simulink library "phasedenvlib"  (R2018b)
settings: Solver=ode45  StartTime=0.0  StopTime=10.0  RelTol=1e-3  EnableMultiTasking=on
undefined symbols (not defined in the file or in its folder): azelaxes, phased, physconst
settings Model: Creator=The MathWorks, Inc.  LastModifiedBy=The MathWorks, Inc.
settings DataIOCC: LimitDataPoints=on  SaveFormat=Array
settings OptimizationCC: LifeSpan=inf
settings DebuggingCC: UnderspecifiedInitializationDetection=Classic  MergeDetectMultiDrivingBlocksExec=none  SolverPrmCheckMsg=warning  AllowSymbolicDim=off  SFUnexpectedBacktrackingDiag=warning  SFNoUnconditionalDefaultTransitionDiag=warning  SFExecutionAtInitializationDiag=none
settings HardwareCC: ProdBitPerPointer=32  ProdBitPerSizeT=32  ProdBitPerPtrDiffT=32  ProdLargestAtomicFloat=None  ProdIntDivRoundTo=Undefined  ProdEndianess=Unspecified  ProdWordSize=32  ProdHWDeviceType=32-bit Generic
settings ModelReferenceCC: PropagateSignalLabelsOutOfModel=off
settings SFSimCC: SimUseLocalCustomCode=off
settings RTWCC: RTWUseLocalCustomCode=off
settings CodeAppCC: StateflowObjectComments=on
settings GRTTargetCC: TargetLangStandard=C89/C90 (ANSI)  GeneratePreprocessorConditionals=Disable all
settings ConfigComp: CovMetricSettings=dw  CovHtmlReporting=on  CovSaveCumulativeToWorkspaceVar=on  CovSaveSingleToWorkspaceVar=on  CovShowResultsExplorer=off  CovExternalEMLEnable=off  CovSFcnEnable=off

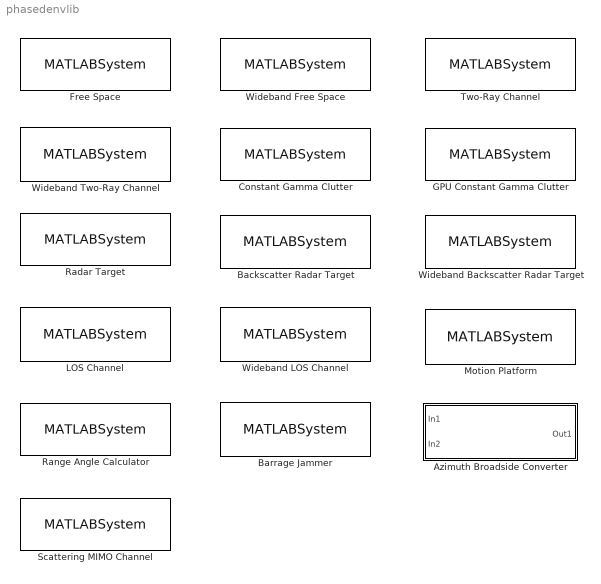
== system phasedenvlib ==
  Azimuth Broadside Converter : Subsystem  VariantControlMode=Label  Variant=on  LabelModeActiveChoice=AzimuthToBroadside  mask(Azimuth/broadside converter){Mode=azimuth -> broadside}
      mask prompts: Mode "Conversion mode:"
      mask help: Conversion between azimuth and broadside angles.
      mask init:
      | modestr = get_param(gcb,'Mode');
      | if modestr(1) == 'a'
      |     mvarctrl = 'AzimuthToBroadside';
      |     inportlabel = 'az';
      |     outportlabel = 'bsd';
      |     titlestr = 'az->bsd';
      | else
      |     mvarctrl = 'BroadsideToAzimuth';
      |     inportlabel = 'bsd';
      |     outportlabel = 'az';
      |     titlestr = 'bsd->az';
      | end
      | set_param(gcb, 'OverrideUsingVariant', mvarctrl);
      mask TypeOptions Mode: azimuth -> broadside | broadside -> azimuth
      mask Display:
      | port_label('input',1,inportlabel);
      | port_label('input',2,'el');
      | port_label('output',1,outportlabel);
      | fprintf('%s',titlestr)
  Backscatter Radar Target : MATLABSystem  System=phased.BackscatterRadarTarget  EnablePolarization=off  AzimuthAngles=-180:180  ElevationAngles=-90:90  RCSPattern=ones(181,361)  ShhPattern=ones(181,361)  ShvPattern=ones(181,361)  SvvPattern=ones(181,361)  Model=Nonfluctuating  PropagationSpeed=physconst( 'LightSpeed' )  OperatingFrequency=3e8  SeedSource=Property  Seed=randi(65535,1)  SimulateUsing=Interpreted execution
      mask Type: phased.BackscatterRadarTarget
      mask Display:
      | disp(['Backscatter' char(10) ' Target']);
      | port_label('input',1,'X');
      | port_label('input',2,'Ang');
  Barrage Jammer : MATLABSystem  System=phased.internal.SimulinkBarrageJammer  ERP=5000  SamplesPerFrameSource=Property  SamplesPerFrame=100  SeedSource=Property  Seed=randi(65535,1)  SimulateUsing=Interpreted execution
      mask Type: phased.internal.SimulinkBarrageJammer
      mask Display: disp('Barrage');
  Constant Gamma Clutter : MATLABSystem  System=phased.internal.SimulinkConstantGammaClutter  Gamma=0  EarthModel=Flat  MaximumRange=5000  AzimuthCoverage=60  PatchAzimuthWidth=1  CoherenceTime=inf  PropagationSpeed=physconst( 'LightSpeed' )  SampleRate=1e6  PRF=1e4  PRFSelectionInputPort=off  SimulationTimeSource=Derive from waveform parameters  OutputFormat=Pulses  NumPulses=1  NumSamples=100  SimulateUsing=Interpreted execution  OperatingFrequency=3e8  TransmitSignalInputPort=off  TransmitERP=5000  PlatformHeight=300  PlatformSpeed=300  PlatformDirection=[ 90; 0 ]  BroadsideDepressionAngle=0  SeedSource=Property  Seed=randi(65535,1)  Sensor=phased.ULA('Element',phased.IsotropicAntennaElement)
      mask Type: phased.internal.SimulinkConstantGammaClutter
      mask Display: disp(['Constant' char(10) 'Gamma Clutter']);
  Free Space : MATLABSystem  System=phased.FreeSpace  PropagationSpeed=physconst( 'LightSpeed' )  OperatingFrequency=3e8  TwoWayPropagation=off  SampleRateFromInputCheckbox=on  SampleRate=1e6  MaximumDistanceSource=Property  MaximumDistance=10e3  MaximumNumInputSamplesSource=Auto  MaximumNumInputSamples=1000  SimulateUsing=Interpreted execution
      mask Type: phased.FreeSpace
      mask Display:
      | disp(['Free Space' char(10) 'Channel']);
      | port_label('input',1,'X');
      | port_label('input',2,'Pos1');
      | port_label('input',3,'Pos2');
      | port_label('input',4,'Vel1');
      | port_label('input',5,'Vel2');
  GPU Constant Gamma Clutter : MATLABSystem  System=phased.gpu.ConstantGammaClutter  Gamma=0  EarthModel=Flat  MaximumRange=5000  AzimuthCoverage=60  PatchAzimuthWidth=1  CoherenceTime=inf  PropagationSpeed=physconst( 'LightSpeed' )  SampleRate=1e6  PRF=1e4  PRFSelectionInputPort=off  OutputFormat=Pulses  NumPulses=1  NumSamples=100  SimulateUsing=Interpreted execution  OperatingFrequency=3e8  TransmitSignalInputPort=off  TransmitERP=5000  PlatformHeight=300  PlatformSpeed=300  PlatformDirection=[ 90; 0 ]  BroadsideDepressionAngle=0  SeedSource=Auto  Seed=0  Sensor=phased.ULA('Element',phased.IsotropicAntennaElement)
      mask Type: phased.gpu.ConstantGammaClutter
      mask Display: disp(['GPU Constant' char(10) 'Gamma Clutter']);
  LOS Channel : MATLABSystem  System=phased.LOSChannel  PropagationSpeed=physconst( 'LightSpeed' )  OperatingFrequency=3e8  SpecifyAtmosphere=off  Temperature=15  DryAirPressure=101325  WaterVapourDensity=7.5  LiquidWaterDensity=0  RainRate=0  TwoWayPropagation=off  SampleRateFromInputCheckbox=on  SampleRate=1e6  MaximumDistanceSource=Property  MaximumDistance=10e3  MaximumNumInputSamplesSource=Auto  MaximumNumInputSamples=1000  SimulateUsing=Interpreted execution
      mask Type: phased.LOSChannel
      mask Display:
      | disp(['LOS' char(10) 'Channel']);
      | port_label('input',1,'X');
      | port_label('input',2,'Pos1');
      | port_label('input',3,'Pos2');
      | port_label('input',4,'Vel1');
      | port_label('input',5,'Vel2');
  Motion Platform : MATLABSystem  System=phased.internal.SimulinkPlatform  MotionModel=Velocity  InitialPosition=[ 0; 0; 0 ]  InitialVelocity=[ 0; 0; 0 ]  VelocitySource=Property  Velocity=[0;0;0]  AccelerationSource=Property  Acceleration=[0;0;0]  CustomTrajectory=[ 0, 0, 0, 0, 0, 0, 0; 1, 0, 0, 0, 0, 0, 0 ]  ScanMode=None  InitialScanAngle=0  AzimuthSpan=[ -60, 60 ]  AzimuthScanRate=10  InitialOrientationAxes=eye( 3 )  OrientationAxesOutputPort=off  ElapsedTimeSource=Auto  SampleRateFromInputCheckbox=on  SampleRate=1e6  SimulateUsing=Interpreted execution
      mask Type: phased.internal.SimulinkPlatform
      mask Display:
      | disp('Platform');
      | port_label('output',1,'Pos');
      | port_label('output',2,'Vel');
  Radar Target : MATLABSystem  System=phased.RadarTarget  EnablePolarization=off  Mode=Monostatic  MeanRCSSource=Property  ScatteringMatrixSource=Property  MeanRCS=1  ScatteringMatrix=eye( 2 )  Model=Nonfluctuating  PropagationSpeed=physconst( 'LightSpeed' )  OperatingFrequency=3e8  SeedSource=Property  Seed=randi(65535,1)  SimulateUsing=Interpreted execution
      mask Type: phased.RadarTarget
      mask Display:
      | disp('Target');
      | port_label('input',1,'X');
  Range Angle Calculator : MATLABSystem  System=phased.internal.RangeAngle  Model=Free space  ReferencePositionSource=Property  ReferencePosition=[ 0; 0; 0 ]  ReferenceAxesSource=Property  ReferenceAxes=eye( 3 )  Output=Angle  SimulateUsing=Interpreted execution
      mask Type: phased.internal.RangeAngle
      mask Display:
      | disp(['Range' char(10) 'Angle']);
      | port_label('input',1,'Pos');
      | port_label('output',1,'Ang');
  Scattering MIMO Channel : MATLABSystem  System=phased.ScatteringMIMOChannel  PropagationSpeed=physconst( 'LightSpeed' )  CarrierFrequency=3e8  Polarization=None  SpecifyAtmosphere=off  Temperature=15  DryAirPressure=101325  WaterVapourDensity=7.5  LiquidWaterDensity=0  RainRate=0  SampleRateFromInputCheckbox=on  SampleRate=1e6  SimulateDirectPath=off  MaximumDelaySource=Property  MaximumDelay=10e-6  ChannelResponseOutputPort=off  SimulateUsing=Interpreted execution  TransmitArray=phased.ULA  ReceiveArray=phased.ULA  TransmitArrayMotionSource=Property  TransmitArrayPosition=[ 0; 0; 0 ]  TransmitArrayOrientationAxes=eye( 3 )  ReceiveArrayMotionSource=Property  ReceiveArrayPosition=[ physconst( 'LightSpeed' )/1e5; 0; 0 ]  ReceiveArrayOrientationAxes=azelaxes( 180, 0 )  ScattererSpecificationSource=Auto  NumScatterers=1  ScattererPositionBoundary=[ 0, 1000 ]  ScattererPosition=[ physconst( 'LightSpeed' )*5e-6; 0; 0 ]  ScattererCoefficient=1  ScatteringMatrix=eye( 2 )  ScattererOrientationAxes=eye( 3 )  SeedSource=Property  Seed=randi(65535,1)
      mask Type: phased.ScatteringMIMOChannel
      mask Display:
      | disp('Scattering\nMIMO Channel');
      | port_label('input',1,'X');
      | port_label('output',1,'Y');
  Two-Ray Channel : MATLABSystem  System=phased.TwoRayChannel  PropagationSpeed=physconst( 'LightSpeed' )  OperatingFrequency=3e8  SpecifyAtmosphere=off  Temperature=15  DryAirPressure=101325  WaterVapourDensity=7.5  LiquidWaterDensity=0  RainRate=0  SampleRateFromInputCheckbox=on  SampleRate=1e6  GroundReflectionCoefficient=-1  GroundRelativePermittivity=15  CombinedRaysOutput=on  MaximumDistanceSource=Property  MaximumDistance=10e3  MaximumNumInputSamplesSource=Auto  MaximumNumInputSamples=1000  SimulateUsing=Interpreted execution
      mask Type: phased.TwoRayChannel
      mask Display:
      | disp(['Two-Ray' char(10) 'Channel']);
      | port_label('input',1,'X');
      | port_label('input',2,'Pos1');
      | port_label('input',3,'Pos2');
      | port_label('input',4,'Vel1');
      | port_label('input',5,'Vel2');
  Wideband Backscatter Radar Target : MATLABSystem  System=phased.WidebandBackscatterRadarTarget  EnablePolarization=off  FrequencyVector=[ 0, 1e20 ]  AzimuthAngles=-180:180  ElevationAngles=-90:90  RCSPattern=ones(181,361)  ShhPattern=ones(181,361)  ShvPattern=ones(181,361)  SvvPattern=ones(181,361)  Model=Nonfluctuating  PropagationSpeed=physconst( 'LightSpeed' )  OperatingFrequency=3e8  SampleRateFromInputCheckbox=on  SampleRate=1e6  NumSubbands=64  SeedSource=Property  Seed=randi(65535,1)  SimulateUsing=Interpreted execution
      mask Type: phased.WidebandBackscatterRadarTarget
      mask Display:
      | disp(['Wideband' char(10) ' Backscatter' char(10) ' Target']);
      | port_label('input',1,'X');
      | port_label('input',2,'Ang');
  Wideband Free Space : MATLABSystem  System=phased.WidebandFreeSpace  PropagationSpeed=physconst( 'LightSpeed' )  OperatingFrequency=3e8  TwoWayPropagation=off  SampleRateFromInputCheckbox=on  SampleRate=1e6  NumSubbands=64  MaximumDistanceSource=Property  MaximumDistance=10e3  MaximumNumInputSamplesSource=Auto  MaximumNumInputSamples=1000  SimulateUsing=Interpreted execution
      mask Type: phased.WidebandFreeSpace
      mask Display:
      | disp(['Wideband' char(10) 'Free Space' char(10) 'Channel']);
      | port_label('input',1,'X');
      | port_label('input',2,'Pos1');
      | port_label('input',3,'Pos2');
      | port_label('input',4,'Vel1');
      | port_label('input',5,'Vel2');
  Wideband LOS Channel : MATLABSystem  System=phased.WidebandLOSChannel  PropagationSpeed=physconst( 'LightSpeed' )  OperatingFrequency=3e8  NumSubbands=64  SpecifyAtmosphere=off  Temperature=15  DryAirPressure=101325  WaterVapourDensity=7.5  LiquidWaterDensity=0  RainRate=0  TwoWayPropagation=off  SampleRateFromInputCheckbox=on  SampleRate=1e6  MaximumDistanceSource=Property  MaximumDistance=10e3  MaximumNumInputSamplesSource=Auto  MaximumNumInputSamples=1000  SimulateUsing=Interpreted execution
      mask Type: phased.WidebandLOSChannel
      mask Display:
      | disp(['Wideband LOS' char(10) 'Channel']);
      | port_label('input',1,'X');
      | port_label('input',2,'Pos1');
      | port_label('input',3,'Pos2');
      | port_label('input',4,'Vel1');
      | port_label('input',5,'Vel2');
  Wideband Two-Ray Channel : MATLABSystem  System=phased.WidebandTwoRayChannel  PropagationSpeed=physconst( 'LightSpeed' )  OperatingFrequency=3e8  NumSubbands=64  SpecifyAtmosphere=off  Temperature=15  DryAirPressure=101325  WaterVapourDensity=7.5  LiquidWaterDensity=0  RainRate=0  SampleRateFromInputCheckbox=on  SampleRate=1e6  GroundReflectionCoefficient=-1  GroundRelativePermittivity=15  CombinedRaysOutput=on  MaximumDistanceSource=Property  MaximumDistance=10e3  MaximumNumInputSamplesSource=Auto  MaximumNumInputSamples=1000  SimulateUsing=Interpreted execution
      mask Type: phased.WidebandTwoRayChannel
      mask Display:
      | disp(['Wideband Two-Ray' char(10) 'Channel']);
      | port_label('input',1,'X');
      | port_label('input',2,'Pos1');
      | port_label('input',3,'Pos2');
      | port_label('input',4,'Vel1');
      | port_label('input',5,'Vel2');

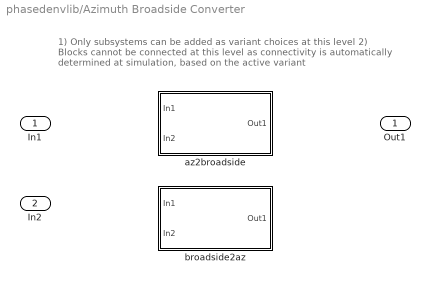
== system phasedenvlib/Azimuth Broadside Converter ==
  note: 1) Only subsystems can be added as variant choices at this level
      | 2) Blocks cannot be connected at this level as connectivity is
      | automatically determined at simulation, based on the active variant
  In1 : Inport
  In2 : Inport  Port=2
  az2broadside : Subsystem  VariantControl=AzimuthToBroadside
  broadside2az : Subsystem  VariantControl=BroadsideToAzimuth
  Out1 : Outport

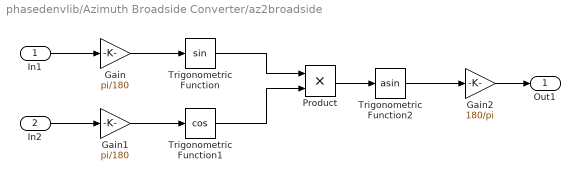
== system phasedenvlib/Azimuth Broadside Converter/az2broadside ==
  In1 : Inport
  In2 : Inport  Port=2
  Gain : Gain  Gain=pi/180
  Gain1 : Gain  Gain=pi/180
  Gain2 : Gain  Gain=180/pi
  Product : Product
  Trigonometric Function : Trigonometry
  Trigonometric Function1 : Trigonometry  Operator=cos
  Trigonometric Function2 : Trigonometry  Operator=asin
  Out1 : Outport
  wires:
  Product/1 -> Trigonometric Function2/1
  Gain2/1 -> Out1/1
  Trigonometric Function1/1 -> Product/2
  Trigonometric Function/1 -> Product/1
  Trigonometric Function2/1 -> Gain2/1
  Gain/1 -> Trigonometric Function/1
  In1/1 -> Gain/1
  In2/1 -> Gain1/1
  Gain1/1 -> Trigonometric Function1/1

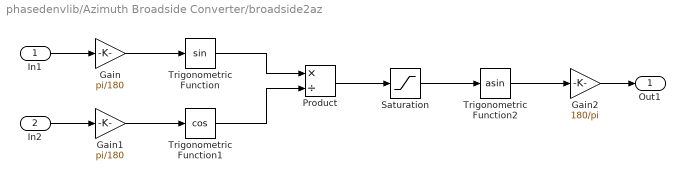
== system phasedenvlib/Azimuth Broadside Converter/broadside2az ==
  In1 : Inport
  In2 : Inport  Port=2
  Gain : Gain  Gain=pi/180
  Gain1 : Gain  Gain=pi/180
  Gain2 : Gain  Gain=180/pi
  Product : Product  Inputs=*/
  Saturation : Saturate  UpperLimit=1  LowerLimit=-1
  Trigonometric Function : Trigonometry
  Trigonometric Function1 : Trigonometry  Operator=cos
  Trigonometric Function2 : Trigonometry  Operator=asin
  Out1 : Outport
  wires:
  Saturation/1 -> Trigonometric Function2/1
  Gain1/1 -> Trigonometric Function1/1
  In2/1 -> Gain1/1
  In1/1 -> Gain/1
  Gain/1 -> Trigonometric Function/1
  Trigonometric Function2/1 -> Gain2/1
  Trigonometric Function/1 -> Product/1
  Trigonometric Function1/1 -> Product/2
  Gain2/1 -> Out1/1
  Product/1 -> Saturation/1
